simulink model "pwm_control"  (R2022a)
settings: Solver=ode4  StartTime=0.0  StopTime=0.1  FixedStep=dt  RelTol=1e-3
values from neighbouring files (symbols this model uses):
  dt = 1e-5    (= 1e-05)    [pwm_fourier_analysis.m]
  Edc = 400    [pwm_fourier_analysis.m]
  fm = 50    [pwm_fourier_analysis.m]
  fs = 1000    [pwm_fourier_analysis.m]
  L = max(size(x))    [Function2Fourier.m]    (also in pwm_fourier_analysis.m = 0.001)
  m = Vr/Edc    (= 0.45)    [pwm_fourier_analysis.m]
  R = 0.01    [pwm_fourier_analysis.m]
  Vr = 180    [pwm_fourier_analysis.m]
libraries: spsControlledVoltageSourceLib x18, spsGroundLib x12, simulink x7, spsThreePhaseParallelRLCBranchLib x6, spsThreePhaseVIMeasurementLib x6, spspowerguiLib x1
settings Model: Creator=msousa2021  LastModifiedBy=marco
settings DebuggingCC: UnconnectedInputMsg=warning  UnconnectedOutputMsg=warning  UnconnectedLineMsg=warning
settings RTWCC: DLArmComputeVersion=19.05

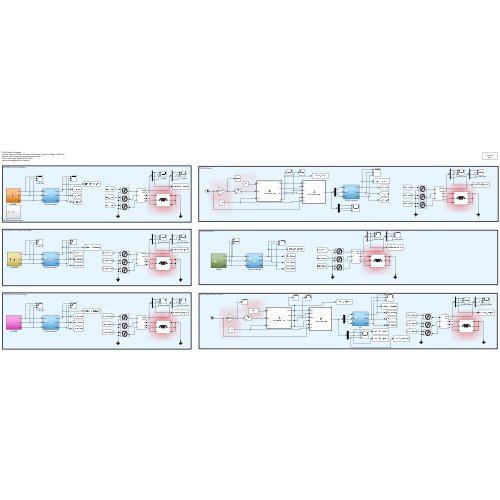
[thumbnail: Simulink's stored preview of the top-level diagram]
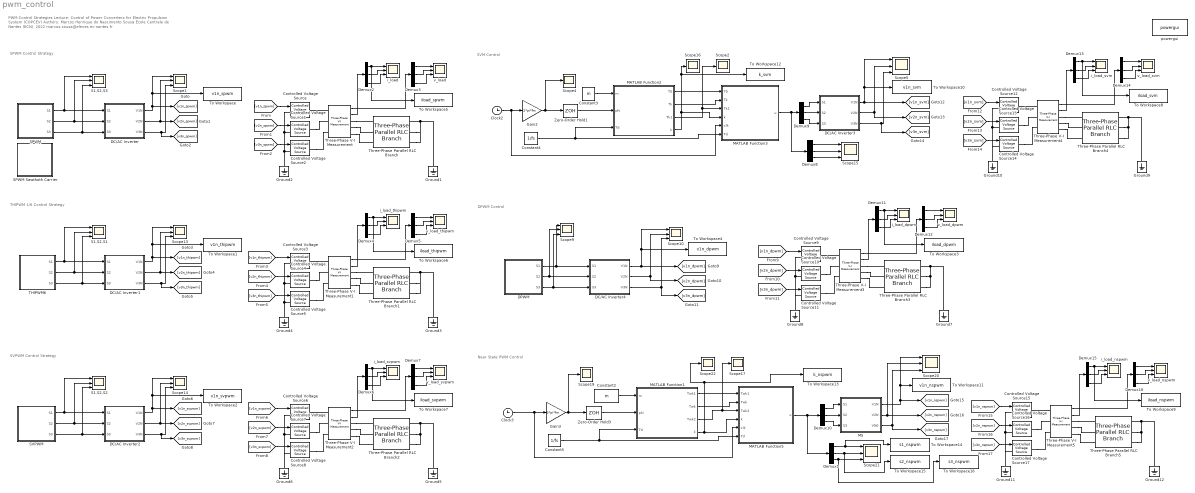
== system pwm_control ==
  note: SPWM Control Strategy
  note: PWM Control Strategies
      | Lecture: Control of Power Converters for Electric Propulsion System (COPCEV)
      | Authors: Marcos Henrique do Nascimento Sousa
      | École Centrale de Nantes (ECN), 2022
      | marcos.sousa@eleves.ec-nantes.fr
  note: THIPWM 1/6 Control Strategy
  note: SVPWM Control Strategy
  note: SVM Control
  note: DPWM Control
  note: Near State PWM Control
  Clock2 : Clock
  Clock3 : Clock
  Constant2 : Constant  Value=m
  Constant3 : Constant  Value=m
  Constant4 : Constant  Value=1/fs
  Constant5 : Constant  Value=1/fs
  Controlled Voltage Source{,1..17} (18 alike) : spsControlledVoltageSourceLib/Controlled Voltage Source  Initialize=on  Source_Type=AC  Amplitude=0  Phase=0  Frequency=0  Measurements=None
  DC/AC Inverter : Subsystem
  DC/AC Inverter1 : Subsystem
  DC/AC Inverter2 : Subsystem
  DC/AC Inverter3 : Subsystem
  DC/AC Inverter4 : Subsystem
  DPWM : Subsystem
  Demux{1..16} (16 alike) : Demux  Outputs=3
  Gain2 : Gain  Gain=2*pi*fm
  Gain3 : Gain  Gain=2*pi*fm
  Ground{1..12} (12 alike) : spsGroundLib/Ground  LConnTagsString=a
  M5 : Subsystem
  MATLAB Function1 : MATLAB Function  TreatAsAtomicUnit=on
  MATLAB Function2 : MATLAB Function  TreatAsAtomicUnit=on
  MATLAB Function3 : MATLAB Function  TreatAsAtomicUnit=on
  MATLAB Function5 : MATLAB Function  TreatAsAtomicUnit=on
  S1,S2,S1 : Scope  NumInputPorts=3
  S1,S2,S2 : Scope  NumInputPorts=3
  S1,S2,S3 : Scope  NumInputPorts=3
  SPWM : Subsystem
  SPWM Sawthoth Carrier : Subsystem
  SVPWM : Subsystem
  Scope{1,5,9..10,13..15,20..21} (9 alike) : Scope  NumInputPorts=3
  Scope{2,4,16..17,19,22} (6 alike) : Scope
  THIPWM6 : Subsystem
  Three-Phase Parallel RLC Branch{,1..5} (6 alike) : spsThreePhaseParallelRLCBranchLib/Three-Phase Parallel RLC Branch  LConnTagsString=A|B|C  RConnTagsString=A|B|C  BranchType=L  Resistance=R  Inductance=L  Capacitance=0  Measurements=None
      settings: SourceProductBaseCode=PS
  Three-Phase V-I Measurement{,1..5} (6 alike) : spsThreePhaseVIMeasurementLib/Three-Phase V-I Measurement  VoltageMeasurement=phase-to-ground  SetLabelV=off  LabelV=Vabc  Vpu=off  VpuLL=off  CurrentMeasurement=yes  SetLabelI=off  LabelI=Iabc  Ipu=off  Pbase=100e6  Vbase=500e3  OutputType=Complex  PhasorSimulation=off  PSBequivalent=0
  To Workspace : ToWorkspace  VariableName=v1n_spwm  SampleTime=-1
      settings: Save2DSignal=2-D array (concatenate along first dimension)
  To Workspace1 : ToWorkspace  VariableName=v1n_thipwm  SampleTime=-1
      settings: Save2DSignal=2-D array (concatenate along first dimension)
  To Workspace10 : ToWorkspace  VariableName=v1n_svm  SampleTime=-1
      settings: Save2DSignal=2-D array (concatenate along first dimension)
  To Workspace11 : ToWorkspace  VariableName=v1n_nspwm  SampleTime=-1
      settings: Save2DSignal=2-D array (concatenate along first dimension)
  To Workspace12 : ToWorkspace  VariableName=k_svm  SampleTime=-1
      settings: Save2DSignal=2-D array (concatenate along first dimension)
  To Workspace13 : ToWorkspace  VariableName=k_nspwm  SampleTime=-1
      settings: Save2DSignal=2-D array (concatenate along first dimension)
  To Workspace14 : ToWorkspace  VariableName=s1_nspwm  SampleTime=-1
      settings: Save2DSignal=2-D array (concatenate along first dimension)
  To Workspace15 : ToWorkspace  VariableName=s2_nspwm  SampleTime=-1
      settings: Save2DSignal=2-D array (concatenate along first dimension)
  To Workspace16 : ToWorkspace  VariableName=s3_nspwm  SampleTime=-1
      settings: Save2DSignal=2-D array (concatenate along first dimension)
  To Workspace2 : ToWorkspace  VariableName=v1n_svpwm  SampleTime=-1
      settings: Save2DSignal=2-D array (concatenate along first dimension)
  To Workspace3 : ToWorkspace  VariableName=iload_dpwm  SampleTime=-1
      settings: Save2DSignal=2-D array (concatenate along first dimension)
  To Workspace4 : ToWorkspace  VariableName=v1n_dpwm  SampleTime=-1
      settings: Save2DSignal=2-D array (concatenate along first dimension)
  To Workspace5 : ToWorkspace  VariableName=iload_spwm  SampleTime=-1
      settings: Save2DSignal=2-D array (concatenate along first dimension)
  To Workspace6 : ToWorkspace  VariableName=iload_thipwm  SampleTime=-1
      settings: Save2DSignal=2-D array (concatenate along first dimension)
  To Workspace7 : ToWorkspace  VariableName=iload_svpwm  SampleTime=-1
      settings: Save2DSignal=2-D array (concatenate along first dimension)
  To Workspace8 : ToWorkspace  VariableName=iload_svm  SampleTime=-1
      settings: Save2DSignal=2-D array (concatenate along first dimension)
  To Workspace9 : ToWorkspace  VariableName=iload_nspwm  SampleTime=-1
      settings: Save2DSignal=2-D array (concatenate along first dimension)
  Zero-Order Hold1 : ZeroOrderHold  SampleTime=-1
  Zero-Order Hold3 : ZeroOrderHold  SampleTime=-1
  i_load : Scope  NumInputPorts=3
  i_load_dpwm : Scope  NumInputPorts=3
  i_load_nspwm : Scope  NumInputPorts=3
  i_load_svm : Scope  NumInputPorts=3
  i_load_svpwm : Scope  NumInputPorts=3
  i_load_thipwm : Scope  NumInputPorts=3
  powergui : spspowerguiLib/powergui  Priority=1  SimulationMode=Discrete  SampleTime=dt  frequency=60  Iterations=50  frequencyindice=0  Pbase=100e6  ErrMax=1e-4  UnitsV=kV  UnitsW=MW  buscounter=0  FunctionMessages=off  echomessages=off  EnableUseOfTLC=off  CurrentSourceSwitches=off  DisableSnubberDevices=off  DisableRonSwitches=off  DisableVfSwitches=off  DisplayEquations=off  AutomaticDiscreteSolvers=off  SolverType=Tustin/Backward Euler (TBE)  Interpol=off  ExternalGateDelay=off  methode=off  Ts=100  x0status=blocks  SPID=on  SwTol=0  HookPort=off  NonlinearTolerance=1e-4  nMaxIteration=100  ContinueOnMaxIteration=off  RestoreLinks=warning  ResistiveCurrentMeasurement=off  Frange=[0:2:500]  Ylog=off  Xlog=on  ShowGrid=off  save=off  variable=ZData  structure=0  ZoomFFT=off  StartTime=0.0  cycles=1  DisplayStyle=1  fundamental=60  FreqAxis=off  MaxFrequency=1000  frequencyindicesteady=1  RmsSteady=1  display=off
  v_load : Scope  NumInputPorts=3
  v_load_dpwm : Scope  NumInputPorts=3
  v_load_nspwm : Scope  NumInputPorts=3
  v_load_svm : Scope  NumInputPorts=3
  v_load_svpwm : Scope  NumInputPorts=3
  v_load_thipwm : Scope  NumInputPorts=3
  wires:
  SPWM/1(S1) -> S1,S2,S3/1, DC/AC Inverter/1(S1)
  SPWM/2(S2) -> S1,S2,S3/2, DC/AC Inverter/2(S2)
  SPWM/3(S3) -> S1,S2,S3/3, DC/AC Inverter/3(S3)
  DC/AC Inverter/1(V1N) -> [v1n_spwm], Scope1/1, To Workspace/1
  DC/AC Inverter/2(V2N) -> [v2n_spwm], Scope1/2
  DC/AC Inverter/3(V3N) -> [v3n_spwm], Scope1/3
  [v1n_spwm] -> Controlled Voltage Source/1
  [v2n_spwm] -> Controlled Voltage Source1/1
  [v3n_spwm] -> Controlled Voltage Source2/1
  Three-Phase V-I Measurement/2 -> Demux2/1
  Demux2/1 -> To Workspace5/1, i_load/1
  Demux2/2 -> i_load/2
  Demux2/3 -> i_load/3
  Demux3/3 -> v_load/3
  Demux3/2 -> v_load/2
  Demux3/1 -> v_load/1
  Three-Phase V-I Measurement/1 -> Demux3/1
  Three-Phase V-I Measurement1/1 -> Demux5/1
  Demux5/1 -> v_load_thipwm/1
  Demux5/2 -> v_load_thipwm/2
  Demux5/3 -> v_load_thipwm/3
  Demux4/3 -> i_load_thipwm/3
  Demux4/2 -> i_load_thipwm/2
  Demux4/1 -> To Workspace6/1, i_load_thipwm/1
  Three-Phase V-I Measurement1/2 -> Demux4/1
  DC/AC Inverter1/3(V3N) -> Scope13/3, [v3n_thipwm]
  DC/AC Inverter1/2(V2N) -> Scope13/2, [v2n_thipwm]
  DC/AC Inverter1/1(V1N) -> To Workspace1/1, Scope13/1, [v1n_thipwm]
  THIPWM6/3(S3) -> DC/AC Inverter1/3(S3), S1,S2,S1/3
  THIPWM6/2(S2) -> DC/AC Inverter1/2(S2), S1,S2,S1/2
  THIPWM6/1(S1) -> DC/AC Inverter1/1(S1), S1,S2,S1/1
  [v1n_thipwm] -> Controlled Voltage Source3/1
  [v2n_thipwm] -> Controlled Voltage Source4/1
  [v3n_thipwm] -> Controlled Voltage Source5/1
  SVPWM/1(S1) -> S1,S2,S2/1, DC/AC Inverter2/1(S1)
  SVPWM/2(S2) -> S1,S2,S2/2, DC/AC Inverter2/2(S2)
  SVPWM/3(S3) -> S1,S2,S2/3, DC/AC Inverter2/3(S3)
  DC/AC Inverter2/1(V1N) -> [v1n_svpwm], Scope14/1, To Workspace2/1
  DC/AC Inverter2/2(V2N) -> [v2n_svpwm], Scope14/2
  DC/AC Inverter2/3(V3N) -> [v3n_svpwm], Scope14/3
  Three-Phase V-I Measurement2/2 -> Demux6/1
  Demux6/1 -> i_load_svpwm/1, To Workspace7/1
  Demux6/2 -> i_load_svpwm/2
  Demux6/3 -> i_load_svpwm/3
  Demux7/3 -> v_load_svpwm/3
  Demux7/2 -> v_load_svpwm/2
  Demux7/1 -> v_load_svpwm/1
  Three-Phase V-I Measurement2/1 -> Demux7/1
  [v1n_svpwm] -> Controlled Voltage Source6/1
  [v2n_svpwm] -> Controlled Voltage Source7/1
  [v3n_svpwm] -> Controlled Voltage Source8/1
  Demux9/2 -> DC/AC Inverter3/2(S2)
  MATLAB Function2/4(k) -> MATLAB Function3/4(k), To Workspace12/1, Scope16/1
  Constant4/1 -> MATLAB Function3/6(Td), MATLAB Function2/3(Td)
  MATLAB Function3/1(u) -> Demux8/1, Demux9/1
  Demux8/2 -> Scope15/2
  MATLAB Function2/2(Tk) -> MATLAB Function3/2(Tk)
  Clock2/1 -> MATLAB Function3/5(clk), Gain2/1
  MATLAB Function2/1(T0) -> MATLAB Function3/1(T0)
  DC/AC Inverter3/1(V1N) -> [v1n_svm], Scope5/1, To Workspace10/1
  Demux8/3 -> Scope15/3
  DC/AC Inverter3/3(V3N) -> [v3n_svm], Scope5/3
  MATLAB Function2/3(Tk1) -> MATLAB Function3/3(Tk1), Scope2/1
  DC/AC Inverter3/2(V2N) -> [v2n_svm], Scope5/2
  Zero-Order Hold1/1 -> MATLAB Function2/2(phi)
  Demux8/1 -> Scope15/1
  Gain2/1 -> Zero-Order Hold1/1, Scope4/1
  Demux9/3 -> DC/AC Inverter3/3(S3)
  Constant3/1 -> MATLAB Function2/1(m)
  Demux9/1 -> DC/AC Inverter3/1(S1)
  DC/AC Inverter4/3(V3N) -> [v3n_dpwm], Scope10/3
  DPWM/2(S2) -> DC/AC Inverter4/2(S2), Scope9/2
  DPWM/3(S3) -> DC/AC Inverter4/3(S3), Scope9/3
  DPWM/1(S1) -> DC/AC Inverter4/1(S1), Scope9/1
  M5/2(V2N) -> Scope20/2, [v2n_nspwm]
  Demux10/1 -> M5/1(S1)
  MATLAB Function1/2(Twk) -> MATLAB Function5/2(Twk)
  Constant2/1 -> MATLAB Function1/1(m)
  Demux10/3 -> M5/3(S3)
  Demux1/2 -> To Workspace15/1, Scope21/2
  M5/3(VN0) -> [v3n_nspwm], Scope20/3
  M5/1(V1N) -> [v1n_nspwm], Scope20/1, To Workspace11/1
  Zero-Order Hold3/1 -> MATLAB Function1/2(phi)
  MATLAB Function5/1(u) -> Demux1/1, Demux10/1
  Demux10/2 -> M5/2(S2)
  Demux1/1 -> To Workspace14/1, Scope21/1
  Gain3/1 -> Zero-Order Hold3/1, Scope19/1
  MATLAB Function1/4(k) -> MATLAB Function5/4(k), Scope22/1, To Workspace13/1
  MATLAB Function1/3(Twk2) -> MATLAB Function5/3(Twk2), Scope17/1
  MATLAB Function1/1(Twk1) -> MATLAB Function5/1(Twk1)
  Constant5/1 -> MATLAB Function5/6(Td), MATLAB Function1/3(Td)
  Clock3/1 -> MATLAB Function5/5(clk), Gain3/1
  Demux12/3 -> v_load_dpwm/3
  [v3n_dpwm] -> Controlled Voltage Source11/1
  [v2n_dpwm] -> Controlled Voltage Source10/1
  Three-Phase V-I Measurement3/2 -> Demux11/1
  [v1n_dpwm] -> Controlled Voltage Source9/1
  Demux11/2 -> i_load_dpwm/2
  Demux12/2 -> v_load_dpwm/2
  Demux12/1 -> v_load_dpwm/1
  Three-Phase V-I Measurement3/1 -> Demux12/1
  Demux11/1 -> To Workspace3/1, i_load_dpwm/1
  Demux11/3 -> i_load_dpwm/3
  DC/AC Inverter4/2(V2N) -> [v2n_dpwm], Scope10/2
  DC/AC Inverter4/1(V1N) -> Scope10/1, To Workspace4/1, [v1n_dpwm]
  [v2n_svm] -> Controlled Voltage Source13/1
  Three-Phase V-I Measurement4/1 -> Demux14/1
  Demux14/2 -> v_load_svm/2
  Demux13/3 -> i_load_svm/3
  Demux14/3 -> v_load_svm/3
  Three-Phase V-I Measurement4/2 -> Demux13/1
  Demux13/2 -> i_load_svm/2
  [v3n_svm] -> Controlled Voltage Source14/1
  [v1n_svm] -> Controlled Voltage Source12/1
  Demux13/1 -> To Workspace8/1, i_load_svm/1
  Demux14/1 -> v_load_svm/1
  [v1n_nspwm] -> Controlled Voltage Source15/1
  [v3n_nspwm] -> Controlled Voltage Source17/1
  Demux15/2 -> i_load_nspwm/2
  Demux16/3 -> v_load_nspwm/3
  Three-Phase V-I Measurement5/2 -> Demux15/1
  Demux16/2 -> v_load_nspwm/2
  Three-Phase V-I Measurement5/1 -> Demux16/1
  Demux15/3 -> i_load_nspwm/3
  [v2n_nspwm] -> Controlled Voltage Source16/1
  Demux15/1 -> To Workspace9/1, i_load_nspwm/1
  Demux16/1 -> v_load_nspwm/1
  Demux1/3 -> To Workspace16/1, Scope21/3
  connections:
  Ground1/LConn1 -- Three-Phase Parallel RLC Branch/RConn3 -- Three-Phase Parallel RLC Branch/RConn2 -- Three-Phase Parallel RLC Branch/RConn1
  Three-Phase V-I Measurement/LConn1 -- Controlled Voltage Source/RConn1
  Controlled Voltage Source1/RConn1 -- Three-Phase V-I Measurement/LConn2
  Controlled Voltage Source2/RConn1 -- Three-Phase V-I Measurement/LConn3
  Three-Phase V-I Measurement/RConn1 -- Three-Phase Parallel RLC Branch/LConn1
  Three-Phase V-I Measurement/RConn2 -- Three-Phase Parallel RLC Branch/LConn2
  Three-Phase V-I Measurement/RConn3 -- Three-Phase Parallel RLC Branch/LConn3
  Controlled Voltage Source2/LConn1 -- Ground2/LConn1 -- Controlled Voltage Source/LConn1 -- Controlled Voltage Source1/LConn1
  Ground3/LConn1 -- Three-Phase Parallel RLC Branch1/RConn1 -- Three-Phase Parallel RLC Branch1/RConn2 -- Three-Phase Parallel RLC Branch1/RConn3
  Controlled Voltage Source5/LConn1 -- Controlled Voltage Source4/LConn1 -- Controlled Voltage Source3/LConn1 -- Ground4/LConn1
  Three-Phase V-I Measurement1/RConn2 -- Three-Phase Parallel RLC Branch1/LConn2
  Controlled Voltage Source4/RConn1 -- Three-Phase V-I Measurement1/LConn2
  Three-Phase V-I Measurement1/LConn1 -- Controlled Voltage Source3/RConn1
  Controlled Voltage Source5/RConn1 -- Three-Phase V-I Measurement1/LConn3
  Three-Phase V-I Measurement1/RConn1 -- Three-Phase Parallel RLC Branch1/LConn1
  Three-Phase V-I Measurement1/RConn3 -- Three-Phase Parallel RLC Branch1/LConn3
  Three-Phase Parallel RLC Branch2/RConn2 -- Ground5/LConn1 -- Three-Phase Parallel RLC Branch2/RConn1 -- Three-Phase Parallel RLC Branch2/RConn3
  Controlled Voltage Source7/LConn1 -- Controlled Voltage Source8/LConn1 -- Ground6/LConn1 -- Controlled Voltage Source6/LConn1
  Three-Phase V-I Measurement2/RConn1 -- Three-Phase Parallel RLC Branch2/LConn1
  Controlled Voltage Source8/RConn1 -- Three-Phase V-I Measurement2/LConn3
  Three-Phase V-I Measurement2/RConn3 -- Three-Phase Parallel RLC Branch2/LConn3
  Three-Phase V-I Measurement2/RConn2 -- Three-Phase Parallel RLC Branch2/LConn2
  Controlled Voltage Source7/RConn1 -- Three-Phase V-I Measurement2/LConn2
  Three-Phase V-I Measurement2/LConn1 -- Controlled Voltage Source6/RConn1
  Controlled Voltage Source9/LConn1 -- Controlled Voltage Source11/LConn1 -- Ground8/LConn1 -- Controlled Voltage Source10/LConn1
  Three-Phase Parallel RLC Branch3/RConn3 -- Ground7/LConn1 -- Three-Phase Parallel RLC Branch3/RConn1 -- Three-Phase Parallel RLC Branch3/RConn2
  Controlled Voltage Source11/RConn1 -- Three-Phase V-I Measurement3/LConn3
  Controlled Voltage Source10/RConn1 -- Three-Phase V-I Measurement3/LConn2
  Three-Phase V-I Measurement3/RConn1 -- Three-Phase Parallel RLC Branch3/LConn1
  Three-Phase V-I Measurement3/RConn3 -- Three-Phase Parallel RLC Branch3/LConn3
  Three-Phase V-I Measurement3/RConn2 -- Three-Phase Parallel RLC Branch3/LConn2
  Three-Phase V-I Measurement3/LConn1 -- Controlled Voltage Source9/RConn1
  Controlled Voltage Source13/LConn1 -- Controlled Voltage Source14/LConn1 -- Ground10/LConn1 -- Controlled Voltage Source12/LConn1
  Three-Phase Parallel RLC Branch4/RConn2 -- Ground9/LConn1 -- Three-Phase Parallel RLC Branch4/RConn1 -- Three-Phase Parallel RLC Branch4/RConn3
  Three-Phase V-I Measurement4/LConn1 -- Controlled Voltage Source12/RConn1
  Three-Phase V-I Measurement4/RConn2 -- Three-Phase Parallel RLC Branch4/LConn2
  Controlled Voltage Source14/RConn1 -- Three-Phase V-I Measurement4/LConn3
  Three-Phase V-I Measurement4/RConn1 -- Three-Phase Parallel RLC Branch4/LConn1
  Controlled Voltage Source13/RConn1 -- Three-Phase V-I Measurement4/LConn2
  Three-Phase V-I Measurement4/RConn3 -- Three-Phase Parallel RLC Branch4/LConn3
  Three-Phase Parallel RLC Branch5/RConn2 -- Three-Phase Parallel RLC Branch5/RConn3 -- Ground12/LConn1 -- Three-Phase Parallel RLC Branch5/RConn1
  Controlled Voltage Source16/LConn1 -- Controlled Voltage Source17/LConn1 -- Ground11/LConn1 -- Controlled Voltage Source15/LConn1
  Three-Phase V-I Measurement5/RConn3 -- Three-Phase Parallel RLC Branch5/LConn3
  Controlled Voltage Source16/RConn1 -- Three-Phase V-I Measurement5/LConn2
  Three-Phase V-I Measurement5/RConn1 -- Three-Phase Parallel RLC Branch5/LConn1
  Controlled Voltage Source17/RConn1 -- Three-Phase V-I Measurement5/LConn3
  Three-Phase V-I Measurement5/LConn1 -- Controlled Voltage Source15/RConn1
  Three-Phase V-I Measurement5/RConn2 -- Three-Phase Parallel RLC Branch5/LConn2

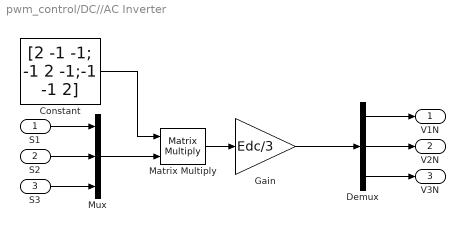
== system pwm_control/DC//AC Inverter ==
  S1 : Inport
  S2 : Inport  Port=2
  S3 : Inport  Port=3
  Constant : Constant  Value=[2 -1 -1; -1 2 -1;-1 -1 2]
  Demux : Demux  Outputs=3
  Gain : Gain  Gain=Edc/3
  Matrix Multiply : Product  Multiplication=Matrix(*)
  Mux : Mux  Inputs=3
  V1N : Outport
  V2N : Outport  Port=2
  V3N : Outport  Port=3
  wires:
  Demux/3 -> V3N/1
  Constant/1 -> Matrix Multiply/1
  S3/1 -> Mux/3
  Matrix Multiply/1 -> Gain/1
  Mux/1 -> Matrix Multiply/2
  S1/1 -> Mux/1
  S2/1 -> Mux/2
  Demux/1 -> V1N/1
  Demux/2 -> V2N/1
  Gain/1 -> Demux/1

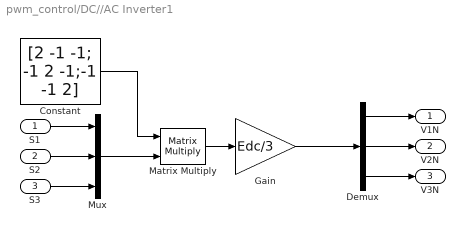
== system pwm_control/DC//AC Inverter1 ==
  S1 : Inport
  S2 : Inport  Port=2
  S3 : Inport  Port=3
  Constant : Constant  Value=[2 -1 -1; -1 2 -1;-1 -1 2]
  Demux : Demux  Outputs=3
  Gain : Gain  Gain=Edc/3
  Matrix Multiply : Product  Multiplication=Matrix(*)
  Mux : Mux  Inputs=3
  V1N : Outport
  V2N : Outport  Port=2
  V3N : Outport  Port=3
  wires:
  Gain/1 -> Demux/1
  Demux/2 -> V2N/1
  Demux/1 -> V1N/1
  S2/1 -> Mux/2
  S1/1 -> Mux/1
  Mux/1 -> Matrix Multiply/2
  Matrix Multiply/1 -> Gain/1
  S3/1 -> Mux/3
  Constant/1 -> Matrix Multiply/1
  Demux/3 -> V3N/1

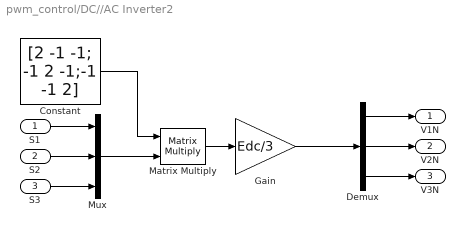
== system pwm_control/DC//AC Inverter2 ==
  S1 : Inport
  S2 : Inport  Port=2
  S3 : Inport  Port=3
  Constant : Constant  Value=[2 -1 -1; -1 2 -1;-1 -1 2]
  Demux : Demux  Outputs=3
  Gain : Gain  Gain=Edc/3
  Matrix Multiply : Product  Multiplication=Matrix(*)
  Mux : Mux  Inputs=3
  V1N : Outport
  V2N : Outport  Port=2
  V3N : Outport  Port=3
  wires:
  Demux/3 -> V3N/1
  Constant/1 -> Matrix Multiply/1
  S3/1 -> Mux/3
  Matrix Multiply/1 -> Gain/1
  Mux/1 -> Matrix Multiply/2
  S1/1 -> Mux/1
  S2/1 -> Mux/2
  Demux/1 -> V1N/1
  Demux/2 -> V2N/1
  Gain/1 -> Demux/1

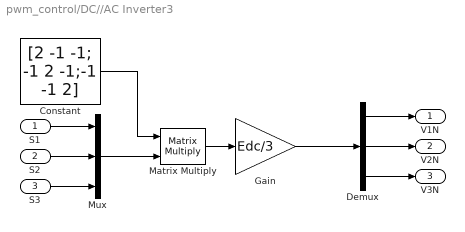
== system pwm_control/DC//AC Inverter3 ==
  S1 : Inport
  S2 : Inport  Port=2
  S3 : Inport  Port=3
  Constant : Constant  Value=[2 -1 -1; -1 2 -1;-1 -1 2]
  Demux : Demux  Outputs=3
  Gain : Gain  Gain=Edc/3
  Matrix Multiply : Product  Multiplication=Matrix(*)
  Mux : Mux  Inputs=3
  V1N : Outport
  V2N : Outport  Port=2
  V3N : Outport  Port=3
  wires:
  Demux/3 -> V3N/1
  Constant/1 -> Matrix Multiply/1
  S3/1 -> Mux/3
  Matrix Multiply/1 -> Gain/1
  Mux/1 -> Matrix Multiply/2
  S1/1 -> Mux/1
  S2/1 -> Mux/2
  Demux/1 -> V1N/1
  Demux/2 -> V2N/1
  Gain/1 -> Demux/1

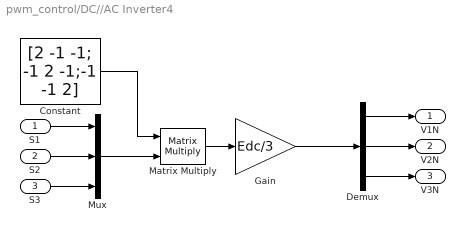
== system pwm_control/DC//AC Inverter4 ==
  S1 : Inport
  S2 : Inport  Port=2
  S3 : Inport  Port=3
  Constant : Constant  Value=[2 -1 -1; -1 2 -1;-1 -1 2]
  Demux : Demux  Outputs=3
  Gain : Gain  Gain=Edc/3
  Matrix Multiply : Product  Multiplication=Matrix(*)
  Mux : Mux  Inputs=3
  V1N : Outport
  V2N : Outport  Port=2
  V3N : Outport  Port=3
  wires:
  Gain/1 -> Demux/1
  Demux/2 -> V2N/1
  Demux/1 -> V1N/1
  S2/1 -> Mux/2
  S1/1 -> Mux/1
  Mux/1 -> Matrix Multiply/2
  Matrix Multiply/1 -> Gain/1
  S3/1 -> Mux/3
  Constant/1 -> Matrix Multiply/1
  Demux/3 -> V3N/1

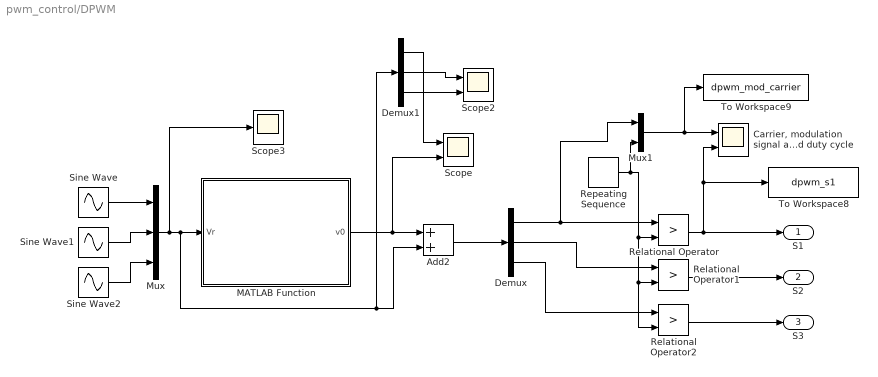
== system pwm_control/DPWM ==
  Add2 : Sum
  "Carrier, modulation signal and duty cycle" : Scope  NumInputPorts=2
  Demux : Demux  Outputs=3
  Demux1 : Demux  Outputs=3
  MATLAB Function : MATLAB Function  TreatAsAtomicUnit=on
  Mux : Mux  Inputs=3
  Mux1 : Mux  Inputs=2
  Relational Operator : RelationalOperator  Operator=>  OutDataTypeStr=boolean  RndMeth=Simplest  InputSameDT=off
  Relational Operator1 : RelationalOperator  Operator=>  OutDataTypeStr=boolean  RndMeth=Simplest  InputSameDT=off
  Relational Operator2 : RelationalOperator  Operator=>  OutDataTypeStr=boolean  RndMeth=Simplest  InputSameDT=off
  Repeating Sequence : simulink/Sources/Repeating Sequence  rep_seq_t=[0; 1/(2*fs); 1/fs]  rep_seq_y=[-0.5; 0.5; -0.5]
  Scope : Scope  NumInputPorts=2
  Scope2 : Scope  NumInputPorts=2
  Scope3 : Scope
  Sine Wave : Sin  Amplitude=m  Frequency=fm*2*pi  SampleTime=0
  Sine Wave1 : Sin  Amplitude=m  Frequency=fm*2*pi  Phase=120*(pi/180)  SampleTime=0
  Sine Wave2 : Sin  Amplitude=m  Frequency=fm*2*pi  Phase=240*(pi/180)  SampleTime=0
  To Workspace8 : ToWorkspace  VariableName=dpwm_s1  SampleTime=-1
      settings: Save2DSignal=2-D array (concatenate along first dimension)
  To Workspace9 : ToWorkspace  VariableName=dpwm_mod_carrier  SampleTime=-1
      settings: Save2DSignal=2-D array (concatenate along first dimension)
  S1 : Outport
  S2 : Outport  Port=2
  S3 : Outport  Port=3
  wires:
  Add2/1 -> Demux/1
  Sine Wave/1 -> Mux/1
  Mux/1 -> Scope3/1, Demux1/1, Add2/2, MATLAB Function/1(Vr)
  Sine Wave1/1 -> Mux/2
  Sine Wave2/1 -> Mux/3
  Demux1/1 -> Scope/1
  Demux1/2 -> Scope2/1
  Demux1/3 -> Scope2/2
  MATLAB Function/1(v0) -> Scope/2, Add2/1
  Mux1/1 -> To Workspace9/1, "Carrier, modulation signal and duty cycle"/1
  Repeating Sequence/1 -> Mux1/2, Relational Operator2/2, Relational Operator1/2, Relational Operator/2
  Relational Operator/1 -> S1/1, To Workspace8/1, "Carrier, modulation signal and duty cycle"/2
  Demux/1 -> Mux1/1, Relational Operator/1
  Demux/2 -> Relational Operator1/1
  Demux/3 -> Relational Operator2/1
  Relational Operator2/1 -> S3/1
  Relational Operator1/1 -> S2/1

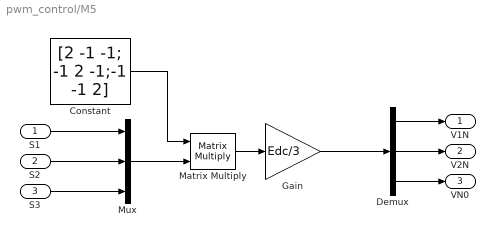
== system pwm_control/M5 ==
  S1 : Inport
  S2 : Inport  Port=2
  S3 : Inport  Port=3
  Constant : Constant  Value=[2 -1 -1; -1 2 -1;-1 -1 2]
  Demux : Demux  Outputs=3
  Gain : Gain  Gain=Edc/3
  Matrix Multiply : Product  Multiplication=Matrix(*)
  Mux : Mux  Inputs=3
  V1N : Outport
  V2N : Outport  Port=2
  VN0 : Outport  Port=3
  wires:
  Demux/3 -> VN0/1
  Constant/1 -> Matrix Multiply/1
  Matrix Multiply/1 -> Gain/1
  Mux/1 -> Matrix Multiply/2
  Demux/1 -> V1N/1
  Demux/2 -> V2N/1
  Gain/1 -> Demux/1
  S1/1 -> Mux/1
  S2/1 -> Mux/2
  S3/1 -> Mux/3

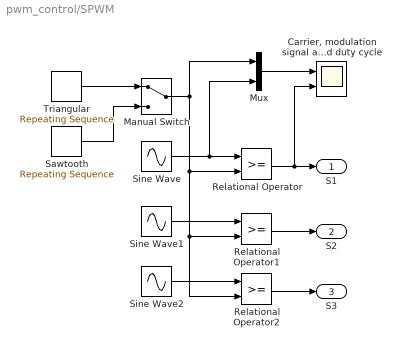
== system pwm_control/SPWM ==
  "Carrier, modulation signal and duty cycle" : Scope  NumInputPorts=2
  Manual Switch : ManualSwitch
  Mux : Mux  Inputs=2
  Relational Operator : RelationalOperator  OutDataTypeStr=boolean  RndMeth=Simplest  InputSameDT=off
  Relational Operator1 : RelationalOperator  OutDataTypeStr=boolean  RndMeth=Simplest  InputSameDT=off
  Relational Operator2 : RelationalOperator  OutDataTypeStr=boolean  RndMeth=Simplest  InputSameDT=off
  Sawtooth : simulink/Sources/Repeating Sequence  rep_seq_t=[0; 1/fs]  rep_seq_y=[-0.5; 0.5]
  Sine Wave : Sin  Amplitude=m  Frequency=fm*2*pi  SampleTime=0
  Sine Wave1 : Sin  Amplitude=m  Frequency=fm*2*pi  Phase=120*(pi/180)  SampleTime=0
  Sine Wave2 : Sin  Amplitude=m  Frequency=fm*2*pi  Phase=240*(pi/180)  SampleTime=0
  Triangular : simulink/Sources/Repeating Sequence  rep_seq_t=[0; 1/(2*fs); 1/fs]  rep_seq_y=[-0.5; 0.5; -0.5]
  S1 : Outport
  S2 : Outport  Port=2
  S3 : Outport  Port=3
  wires:
  Relational Operator2/1 -> S3/1
  Sine Wave/1 -> Mux/2, Relational Operator/1
  Relational Operator/1 -> "Carrier, modulation signal and duty cycle"/2, S1/1
  Relational Operator1/1 -> S2/1
  Sine Wave1/1 -> Relational Operator1/1
  Sine Wave2/1 -> Relational Operator2/1
  Mux/1 -> "Carrier, modulation signal and duty cycle"/1
  Triangular/1 -> Manual Switch/1
  Manual Switch/1 -> Relational Operator2/2, Relational Operator1/2, Relational Operator/2, Mux/1
  Sawtooth/1 -> Manual Switch/2

== system pwm_control/SPWM Sawthoth Carrier ==
  DC/AC Inverter3 : Subsystem
  S1,S2,S4 : Scope  NumInputPorts=3
  SPWM1 : Subsystem
  Scope2 : Scope  NumInputPorts=3
  To Workspace5 : ToWorkspace  VariableName=v1n_spwm_sawtooth  SampleTime=-1
      settings: Save2DSignal=2-D array (concatenate along first dimension)
  wires:
  SPWM1/3(S3) -> DC/AC Inverter3/3(S3), S1,S2,S4/3
  SPWM1/2(S2) -> DC/AC Inverter3/2(S2), S1,S2,S4/2
  SPWM1/1(S1) -> DC/AC Inverter3/1(S1), S1,S2,S4/1
  DC/AC Inverter3/1(V1N) -> To Workspace5/1, Scope2/1
  DC/AC Inverter3/2(V2N) -> Scope2/2
  DC/AC Inverter3/3(V3N) -> Scope2/3

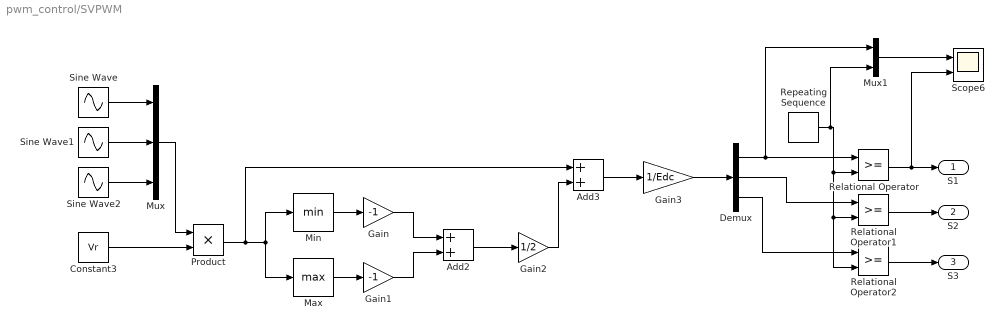
== system pwm_control/SVPWM ==
  Add2 : Sum
  Add3 : Sum
  Constant3 : Constant  Value=Vr
  Demux : Demux  Outputs=3
  Gain : Gain  Gain=-1
  Gain1 : Gain  Gain=-1
  Gain2 : Gain  Gain=1/2
  Gain3 : Gain  Gain=1/Edc
  Max : MinMax  Function=max
  Min : MinMax
  Mux : Mux  Inputs=3
  Mux1 : Mux  Inputs=2
  Product : Product
  Relational Operator : RelationalOperator  OutDataTypeStr=boolean  RndMeth=Simplest  InputSameDT=off
  Relational Operator1 : RelationalOperator  OutDataTypeStr=boolean  RndMeth=Simplest  InputSameDT=off
  Relational Operator2 : RelationalOperator  OutDataTypeStr=boolean  RndMeth=Simplest  InputSameDT=off
  Repeating Sequence : simulink/Sources/Repeating Sequence  rep_seq_t=[0; 1/(2*fs); 1/fs]  rep_seq_y=[-0.5; 0.5; -0.5]
  Scope6 : Scope  NumInputPorts=2
  Sine Wave : Sin  Frequency=fm*2*pi  SampleTime=0
  Sine Wave1 : Sin  Frequency=fm*2*pi  Phase=120*(pi/180)  SampleTime=0
  Sine Wave2 : Sin  Frequency=fm*2*pi  Phase=240*(pi/180)  SampleTime=0
  S1 : Outport
  S2 : Outport  Port=2
  S3 : Outport  Port=3
  wires:
  Demux/3 -> Relational Operator2/1
  Demux/2 -> Relational Operator1/1
  Demux/1 -> Relational Operator/1, Mux1/1
  Relational Operator2/1 -> S3/1
  Relational Operator1/1 -> S2/1
  Relational Operator/1 -> S1/1, Scope6/2
  Repeating Sequence/1 -> Relational Operator2/2, Relational Operator1/2, Relational Operator/2, Mux1/2
  Mux1/1 -> Scope6/1
  Mux/1 -> Product/1
  Constant3/1 -> Product/2
  Sine Wave2/1 -> Mux/3
  Sine Wave1/1 -> Mux/2
  Sine Wave/1 -> Mux/1
  Product/1 -> Add3/1, Max/1, Min/1
  Min/1 -> Gain/1
  Max/1 -> Gain1/1
  Gain/1 -> Add2/1
  Gain1/1 -> Add2/2
  Add2/1 -> Gain2/1
  Gain2/1 -> Add3/2
  Add3/1 -> Gain3/1
  Gain3/1 -> Demux/1

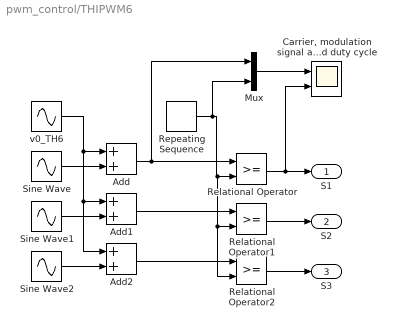
== system pwm_control/THIPWM6 ==
  Add : Sum
  Add1 : Sum
  Add2 : Sum
  "Carrier, modulation signal and duty cycle" : Scope  NumInputPorts=2
  Mux : Mux  Inputs=2
  Relational Operator : RelationalOperator  OutDataTypeStr=boolean  RndMeth=Simplest  InputSameDT=off
  Relational Operator1 : RelationalOperator  OutDataTypeStr=boolean  RndMeth=Simplest  InputSameDT=off
  Relational Operator2 : RelationalOperator  OutDataTypeStr=boolean  RndMeth=Simplest  InputSameDT=off
  Repeating Sequence : simulink/Sources/Repeating Sequence  rep_seq_t=[0; 1/(2*fs); 1/fs]  rep_seq_y=[-0.5; 0.5; -0.5]
  Sine Wave : Sin  Amplitude=m  Frequency=fm*2*pi  SampleTime=0
  Sine Wave1 : Sin  Amplitude=m  Frequency=fm*2*pi  Phase=120*(pi/180)  SampleTime=0
  Sine Wave2 : Sin  Amplitude=m  Frequency=fm*2*pi  Phase=240*(pi/180)  SampleTime=0
  v0_TH6 : Sin  Amplitude=m/6  Frequency=3*fm*2*pi  SampleTime=0
  S1 : Outport
  S2 : Outport  Port=2
  S3 : Outport  Port=3
  wires:
  Relational Operator2/1 -> S3/1
  Relational Operator/1 -> "Carrier, modulation signal and duty cycle"/2, S1/1
  Relational Operator1/1 -> S2/1
  Sine Wave2/1 -> Add2/2
  Sine Wave1/1 -> Add1/2
  Sine Wave/1 -> Add/2
  v0_TH6/1 -> Add2/1, Add1/1, Add/1
  Mux/1 -> "Carrier, modulation signal and duty cycle"/1
  Add/1 -> Mux/1, Relational Operator/1
  Add1/1 -> Relational Operator1/1
  Add2/1 -> Relational Operator2/1
  Repeating Sequence/1 -> Mux/2, Relational Operator2/2, Relational Operator1/2, Relational Operator/2

== system pwm_control/SPWM Sawthoth Carrier/DC//AC Inverter3 ==
  S1 : Inport
  S2 : Inport  Port=2
  S3 : Inport  Port=3
  Constant : Constant  Value=[2 -1 -1; -1 2 -1;-1 -1 2]
  Demux : Demux  Outputs=3
  Gain : Gain  Gain=Edc/3
  Matrix Multiply : Product  Multiplication=Matrix(*)
  Mux : Mux  Inputs=3
  V1N : Outport
  V2N : Outport  Port=2
  V3N : Outport  Port=3
  wires:
  Gain/1 -> Demux/1
  Demux/2 -> V2N/1
  Demux/1 -> V1N/1
  S2/1 -> Mux/2
  S1/1 -> Mux/1
  Mux/1 -> Matrix Multiply/2
  Matrix Multiply/1 -> Gain/1
  S3/1 -> Mux/3
  Constant/1 -> Matrix Multiply/1
  Demux/3 -> V3N/1

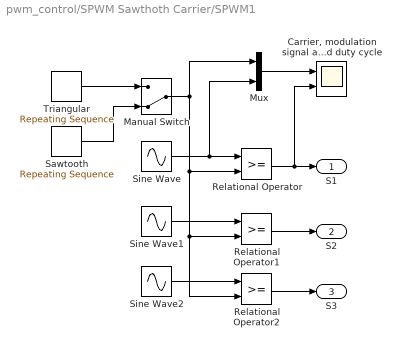
== system pwm_control/SPWM Sawthoth Carrier/SPWM1 ==
  "Carrier, modulation signal and duty cycle" : Scope  NumInputPorts=2
  Manual Switch : ManualSwitch  CurrentSetting=0
  Mux : Mux  Inputs=2
  Relational Operator : RelationalOperator  OutDataTypeStr=boolean  RndMeth=Simplest  InputSameDT=off
  Relational Operator1 : RelationalOperator  OutDataTypeStr=boolean  RndMeth=Simplest  InputSameDT=off
  Relational Operator2 : RelationalOperator  OutDataTypeStr=boolean  RndMeth=Simplest  InputSameDT=off
  Sawtooth : simulink/Sources/Repeating Sequence  rep_seq_t=[0; 1/fs]  rep_seq_y=[-0.5; 0.5]
  Sine Wave : Sin  Amplitude=m  Frequency=fm*2*pi  SampleTime=0
  Sine Wave1 : Sin  Amplitude=m  Frequency=fm*2*pi  Phase=120*(pi/180)  SampleTime=0
  Sine Wave2 : Sin  Amplitude=m  Frequency=fm*2*pi  Phase=240*(pi/180)  SampleTime=0
  Triangular : simulink/Sources/Repeating Sequence  rep_seq_t=[0; 1/(2*fs); 1/fs]  rep_seq_y=[-0.5; 0.5; -0.5]
  S1 : Outport
  S2 : Outport  Port=2
  S3 : Outport  Port=3
  wires:
  Sawtooth/1 -> Manual Switch/2
  Manual Switch/1 -> Mux/1, Relational Operator/2, Relational Operator1/2, Relational Operator2/2
  Triangular/1 -> Manual Switch/1
  Mux/1 -> "Carrier, modulation signal and duty cycle"/1
  Sine Wave2/1 -> Relational Operator2/1
  Sine Wave1/1 -> Relational Operator1/1
  Relational Operator1/1 -> S2/1
  Relational Operator/1 -> S1/1, "Carrier, modulation signal and duty cycle"/2
  Sine Wave/1 -> Relational Operator/1, Mux/2
  Relational Operator2/1 -> S3/1

== matlab function pwm_control/DPWM/MATLAB Function ==
  data: v0 output; Vr input
function v0  = Conduction(Vr)

%a = 1 - 0.5*(1+sign(sin(3*(theta+delta))));
%v0 = 0.5*(1-2*a)+(a-1)*max(Vr)-a*min(Vr);
v0 = -(min(Vr)+1/2);

end

== matlab function pwm_control/MATLAB Function2 ==
  data: m input; T0 output; phi input; Td input; Tk output; Tk1 output; k output
function [T0,Tk,Tk1,k] = ConductionTime(m,phi,Td)

%phi = mod(phi,2*pi);
k = 1+floor(mod(6*phi/(2*pi),6));
% if (phi<60*(pi/180))
%         k = 1;
% elseif (phi>=60*(pi/180) && phi<120*(pi/180))
%         k = 2;
% elseif (phi>=120*(pi/180) && phi<180*(pi/180))
%         k = 3;
% elseif (phi>=180*(pi/180) && phi<240*(pi/180))
%         k = 4;
% elseif (phi>=240*(pi/180) && phi<300*(pi/180))
%         k = 5;
% else %(phi>=300*(pi/180))
%         k = 6;
%     end
    
Tk = sqrt(3)*m*Td*cos(phi+(3-2*k)*pi/6);
Tk1 = sqrt(3)*m*Td*sin(phi+(2-2*k)*pi/6);
T0 = (Td/2)*(1-sqrt(3)*m*cos(phi-(2*k-1)*pi/6));
end

== matlab function pwm_control/MATLAB Function3 ==
  data: T0 input; u output; Tk input; Tk1 input; k input; clk input; Td input
function u  = Time2Switches(T0,Tk,Tk1,k,clk,Td)

clk = mod(clk, 2*Td);

S  = [(clk >= T0) - (clk > ((2*Td)-T0));...
      (clk >= (T0+Tk)) - (clk > ((2*Td)-(T0+Tk)));...
      (clk >= (T0+Tk+Tk1)) - (clk > ((2*Td)-(T0+Tk+Tk1)))];

% Sector 1-6
u =  (k==1)*[S(1),S(2),S(3)] + ...
     (k==2)*[S(2),S(1),S(3)] + ...
     (k==3)*[S(3),S(1),S(2)] + ...
     (k==4)*[S(3),S(2),S(1)] + ...
     (k==5)*[S(2),S(3),S(1)] + ...
     (k==6)*[S(1),S(3),S(2)] ;

%{
sv = [0 0 0; 0 0 1; 0 1 0; 0 1 1; 1 0 0; 1 0 1; 1 1 0; 1 1 1];
%k_period = ["Ts0" "Ts1" "Ts2" "Ts3" "Ts4" "Ts5" "Ts6" "Ts7"];
%d = dictionary(k_period, sequence);
t = mod(clk,2*Td);

if (k ==1)
    sequence = [sv(1,:); sv(5,:); sv(7,:); sv(8,:); sv(8,:); sv(7,:); sv(5,:); sv(1,:)];
elseif (k == 2)
    sequence = [sv(1,:); sv(3,:); sv(7,:); sv(8,:); sv(8,:); sv(7,:); sv(3,:); sv(1,:)];
elseif (k == 3)
    sequence = [sv(1,:); sv(3,:); sv(4,:); sv(8,:); sv(8,:); sv(4,:); sv(3,:); sv(1,:)];
elseif (k == 4)
    sequence = [sv(1,:); sv(2,:); sv(4,:); sv(8,:); sv(8,:); sv(4,:); sv(2,:); sv(1,:)]; 
elseif (k == 5)
    sequence = [sv(1,:); sv(2,:); sv(6,:); sv(8,:); sv(8,:); sv(6,:); sv(2,:); sv(1,:)];
else% (k == 6)
    sequence = [sv(1,:); sv(5,:); sv(6,:); sv(8,:); sv(8,:); sv(6,:); sv(5,:); sv(1,:)];
%else sequence = [sv(1,:); sv(5,:); sv(7,:); sv(8,:); sv(8,:); sv(7,:); sv(5,:); sv(1,:)];
end

if (mod(k,2)==1)
    if (t<T0)
        u = sequence(1,:);
    elseif (t>=T0 && t<(Tk+T0))
        u = sequence(2,:);
    elseif (t>=(Tk+T0) && t<(Td-T0))
        u = sequence(3,:);
    elseif (t>=(Td-T0) && t<Td)
        u = sequence(4,:);
    elseif (t>=(Td) && t<(Td+T0))
        u = sequence(5,:);
    elseif (t>=(Td+T0) && t<(Td+T0+Tk))
        u = sequence(6,:);
    elseif (t>=(Td+T0+Tk) && t<(2*Td-T0))
        u = sequence(7,:);
    else %(t>=(2*Td-T0) && t<(2*Td))
        u = sequence(8,:);
    %else u = sequence(1,:);
    end
else
     if (t<T0)
        u = sequence(1,:);
     elseif (t>=T0 && t<(Tk1+T0))
        u = sequence(2,:);
     elseif (t>=(Tk1+T0) && t<(Td-T0))
        u = sequence(3,:);
     elseif (t>=(Td-T0) && t<Td)
        u = sequence(4,:);
     elseif (t>=(Td) && t<(Td+T0))
        u = sequence(5,:);
     elseif (t>=(Td+T0) && t<(Td+T0+Tk1))
        u = sequence(6,:);
     elseif (t>=(Td+T0+Tk1) && t<(2*Td-T0))
        u = sequence(7,:);
     else %(t>=(2*Td-T0) && t<(2*Td))
        u = sequence(8,:);
        %else u = sequence(1,:);
    end
end
%}

== matlab function pwm_control/MATLAB Function1 ==
  data: m input; Twk1 output; phi input; Td input; Twk output; Twk2 output; k output
function [Twk1,Twk,Twk2,k] = ConductionTime(m,phi,Td)

%phi = mod(phi,2*pi);
k = 1+floor(mod(6*(phi+pi/6)/(2*pi),6));


Twk1 = Td*(1-(sqrt(3)*m)*sin(phi-((k-2)*pi)/3));
Twk = Td*(-1+0.5*(3*m)*(cos(phi-((k-2)*pi)/3)+sqrt(3)*sin(phi-((k-2)*pi)/3)));
Twk2 = Td*(1-0.5*(sqrt(3)*m)*(sqrt(3)*cos(phi-((k-2)*pi)/3)+sin(phi-((k-2)*pi)/3)));

%Twk1 = Td*(1-((2*sqrt(3)*m)/pi)*sin(phi-((k-2)*pi)/3));
%Twk = Td*(-1+(1/pi)*(3*m)*(cos(phi-((k-2)*pi)/3)+sqrt(3)*sin(phi-((k-2)*pi)/3)));
%Twk2 = Td*(1-(1/pi)*(sqrt(3)*m)*(sqrt(3)*cos(phi-((k-2)*pi)/3)+sin(phi-((k-2)*pi)/3)));
end

== matlab function pwm_control/MATLAB Function5 ==
  data: Twk1 input; u output; Twk input; Twk2 input; k input; clk input; Td input
function u  = Time2Switches(Twk1,Twk,Twk2,k,clk,Td)
clk = mod(clk, 2*Td);

S  = [(clk >= Twk2) - (clk > ((2*Td)-Twk2));...
      not((clk > (Twk2+Twk)) - (clk >= ((2*Td)-(Twk2+Twk))));...
      0];

% Sector 1-6
u =  (k==1)*[S(1),S(2),S(3)] + ...
     (k==2)*[S(2),S(1),S(3)] + ...
     (k==3)*[S(3),S(1),S(2)] + ...
     (k==4)*[S(3),S(2),S(1)] + ...
     (k==5)*[S(2),S(3),S(1)] + ...
     (k==6)*[S(1),S(3),S(2)] ;

%{
sv = [0 0 0; 0 0 1; 0 1 0; 0 1 1; 1 0 0; 1 0 1; 1 1 0; 1 1 1];
%k_period = ["Ts0" "Ts1" "Ts2" "Ts3" "Ts4" "Ts5" "Ts6" "Ts7"];
%d = dictionary(k_period, sequence);
t = mod(clk,2*Td);

if (k ==1)
    sequence = [sv(1,:); sv(5,:); sv(7,:); sv(8,:); sv(8,:); sv(7,:); sv(5,:); sv(1,:)];
elseif (k == 2)
    sequence = [sv(1,:); sv(3,:); sv(7,:); sv(8,:); sv(8,:); sv(7,:); sv(3,:); sv(1,:)];
elseif (k == 3)
    sequence = [sv(1,:); sv(3,:); sv(4,:); sv(8,:); sv(8,:); sv(4,:); sv(3,:); sv(1,:)];
elseif (k == 4)
    sequence = [sv(1,:); sv(2,:); sv(4,:); sv(8,:); sv(8,:); sv(4,:); sv(2,:); sv(1,:)]; 
elseif (k == 5)
    sequence = [sv(1,:); sv(2,:); sv(6,:); sv(8,:); sv(8,:); sv(6,:); sv(2,:); sv(1,:)];
else% (k == 6)
    sequence = [sv(1,:); sv(5,:); sv(6,:); sv(8,:); sv(8,:); sv(6,:); sv(5,:); sv(1,:)];
%else sequence = [sv(1,:); sv(5,:); sv(7,:); sv(8,:); sv(8,:); sv(7,:); sv(5,:); sv(1,:)];
end

if (mod(k,2)==1)
    if (t<Twk1)
        u = sequence(1,:);
    elseif (t>=Twk1 && t<(Twk+Twk1))
        u = sequence(2,:);
    elseif (t>=(Twk+Twk1) && t<(Td-Twk1))
        u = sequence(3,:);
    elseif (t>=(Td-Twk1) && t<Td)
        u = sequence(4,:);
    elseif (t>=(Td) && t<(Td+Twk1))
        u = sequence(5,:);
    elseif (t>=(Td+Twk1) && t<(Td+Twk1+Twk))
        u = sequence(6,:);
    elseif (t>=(Td+Twk1+Twk) && t<(2*Td-Twk1))
        u = sequence(7,:);
    elseif (t>=(2*Td-Twk1) && t<(2*Td))
        u = sequence(8,:);
    else u = sequence(1,:);
    end
else
     if (t<Twk1)
        u = sequence(1,:);
    elseif (t>=Twk1 && t<(Twk2+Twk1))
        u = sequence(2,:);
    elseif (t>=(Twk2+Twk1) && t<(Td-Twk1))
        u = sequence(3,:);
    elseif (t>=(Td-Twk1) && t<Td)
        u = sequence(4,:);
    elseif (t>=(Td) && t<(Td+Twk1))
        u = sequence(5,:);
    elseif (t>=(Td+Twk1) && t<(Td+Twk+Twk2))
        u = sequence(6,:);
    elseif (t>=(Td+Twk1+Twk2) && t<(2*Td-Twk1))
        u = sequence(7,:);
    elseif (t>=(2*Td-Twk1) && t<(2*Td))
        u = sequence(8,:);
        else u = sequence(1,:);
    end
end
%}
